simulink model "model1"  (R2025b)
settings: Solver=VariableStepDiscrete  StartTime=0.0  StopTime=inf  MaxStep=0.01  RelTol=1e-3
settings Model: Creator=mammadoo  LastModifiedBy=mammadoo

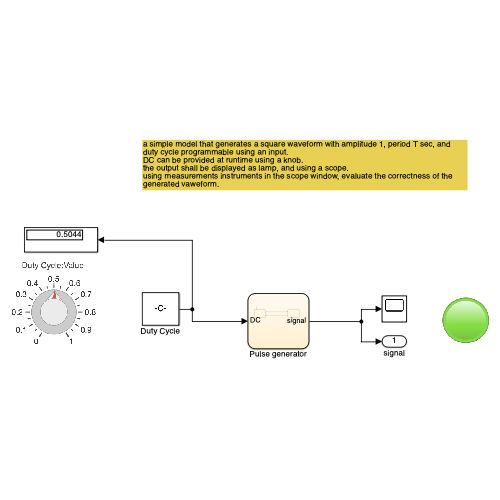
[thumbnail: Simulink's stored preview of the top-level diagram]
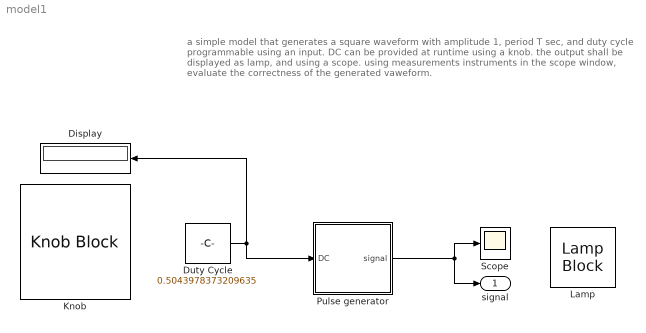
== system model1 ==
  note: a simple model that generates a square waveform with amplitude 1, period T sec, and duty cycle programmable using an input.
      | DC can be provided at runtime using a knob.
      | the output shall be displayed as lamp, and using a scope.
      | using measurements instruments in the scope window, evaluate the correctness of the generated vaweform.
  Display : Display
  Duty Cycle : Constant  Value=0.5043978373209635
  Knob : KnobBlock  ScaleMax=1  TickInterval=0.1
  Lamp : LampBlock  LabelPosition=Hide  DefaultColor=[192.0, 192.0, 192.0]
  Pulse generator : Stateflow chart  TreatAsAtomicUnit=on
  Scope : Scope
      settings: ActiveDisplayYMinimum=-0.12499999999999997  ActiveDisplayYMaximum=1.125
  signal : Outport
  wires:
  Pulse generator/1(signal) -> Scope/1, signal/1
  Duty Cycle/1 -> Display/1, Pulse generator/1(DC)

== stateflow chart model1/Pulse generator ==
  state OFF
    entry:
    signal = 0;
  state ON
    entry:
    signal = 1;
  note: If we check the Simulink solver step size, we observe that it is 0.2
      | so assume that T=1 and DC=50%, when we are in the OFF state and simulation time is 0.2, 0.4 we still stay in the same statesince it will change its state when the sim time is greater than (1-DC)*T. So in the next time stem when the sim time becomes 0.6, it will change its state.
      | here, after doing model-in-the-loop testing, we can claim that the problem is not related to the model and it is due to the solver configuration.
  (default) -> OFF
  OFF -> ON : after((1-DC)*T, sec)
  ON -> OFF : after(DC*T, sec)
  data: signal output; DC input; T constant double =1
